simulink model "feedback_3D"  (R2022a)
settings: Solver=VariableStepAuto  StartTime=0.0  StopTime=10.0  RelTol=1e-3
undefined symbols (not defined in the file): A, B, C, F, G, H, K
settings Model: Creator=Orkun  LastModifiedBy=Orkun

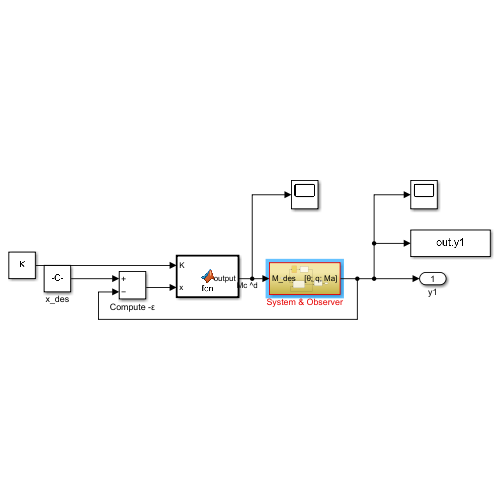
[thumbnail: Simulink's stored preview of the top-level diagram]
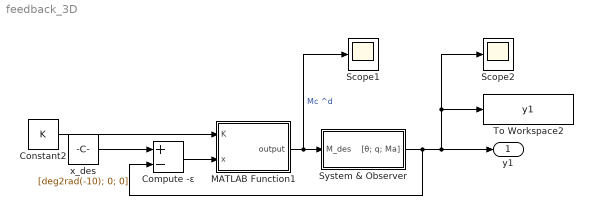
== system feedback_3D ==
  Compute -ε : Sum  Inputs=+-
  Constant2 : Constant  Value=K  VectorParams1D=off
  MATLAB Function1 : MATLAB Function  TreatAsAtomicUnit=on
  Scope1 : Scope
  Scope2 : Scope
  System & Observer : Subsystem
  To Workspace2 : ToWorkspace  VariableName=y1  SaveFormat=Timeseries  SampleTime=-1
  x_des : Constant  Value=[deg2rad(-10); 0; 0]
  y1 : Outport
  wires:
  Compute -ε/1 -> MATLAB Function1/2(x)
  MATLAB Function1/1(output) -> System & Observer/1(M_des), Scope1/1  "Mc ^d"
  Constant2/1 -> MATLAB Function1/1(K)
  x_des/1 -> Compute -ε/1
  System & Observer/1("[θ; q; Ma]") -> Compute -ε/2, Scope2/1, To Workspace2/1, y1/1

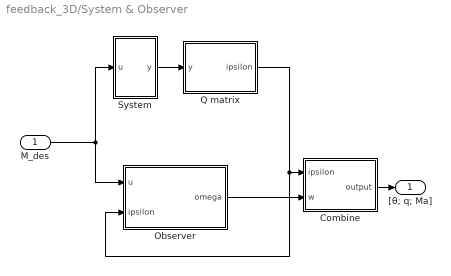
== system feedback_3D/System & Observer ==
  M_des : Inport
  Combine : MATLAB Function  TreatAsAtomicUnit=on
  Observer : Subsystem
  Q matrix : MATLAB Function  TreatAsAtomicUnit=on
  System : Subsystem
  "[θ; q; Ma]" : Outport
  wires:
  M_des/1 -> Observer/1(u), System/1(u)
  Q matrix/1(ipsilon) -> Combine/1(ipsilon), Observer/2(ipsilon)
  Combine/1(output) -> "[θ; q; Ma]"/1
  System/1(y) -> Q matrix/1(y)
  Observer/1(omega) -> Combine/2(w)

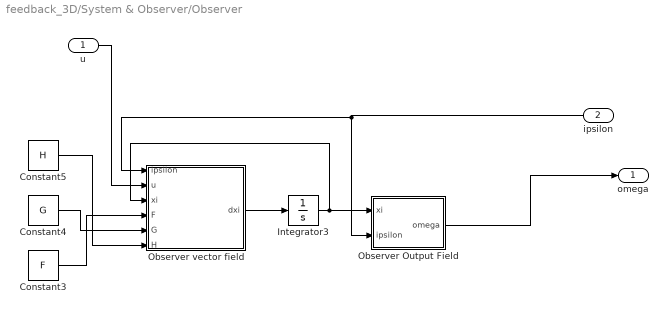
== system feedback_3D/System & Observer/Observer ==
  u : Inport
  ipsilon : Inport  Port=2
  Constant3 : Constant  Value=F
  Constant4 : Constant  Value=G
  Constant5 : Constant  Value=H
  Integrator3 : Integrator  InitialCondition=[0]
  Observer Output Field : MATLAB Function  TreatAsAtomicUnit=on
  Observer vector field : MATLAB Function  TreatAsAtomicUnit=on
  omega : Outport
  wires:
  u/1 -> Observer vector field/2(u)
  Integrator3/1 -> Observer vector field/3(xi), Observer Output Field/1(xi)
  ipsilon/1 -> Observer Output Field/2(ipsilon), Observer vector field/1(ipsilon)
  Constant5/1 -> Observer vector field/6(H)
  Observer Output Field/1(omega) -> omega/1
  Observer vector field/1(dxi) -> Integrator3/1
  Constant4/1 -> Observer vector field/5(G)
  Constant3/1 -> Observer vector field/4(F)

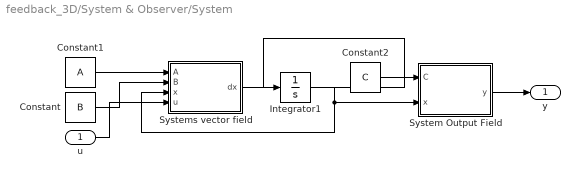
== system feedback_3D/System & Observer/System ==
  u : Inport
  Constant : Constant  Value=B
  Constant1 : Constant  Value=A
  Constant2 : Constant  Value=C
  Integrator1 : Integrator  InitialCondition=[deg2rad(0);0; 0]
  System Output Field : MATLAB Function  TreatAsAtomicUnit=on
  Systems vector field : MATLAB Function  TreatAsAtomicUnit=on
  y : Outport
  wires:
  Systems vector field/1(dx) -> Integrator1/1
  Constant1/1 -> Systems vector field/1(A)
  Constant2/1 -> System Output Field/1(C)
  u/1 -> Systems vector field/4(u)
  Integrator1/1 -> Systems vector field/3(x), System Output Field/2(x)
  System Output Field/1(y) -> y/1
  Constant/1 -> Systems vector field/2(B)

== matlab function feedback_3D/MATLAB Function1 ==
  data: K input; output output; x input
function output = fcn(K, x)

output = K*x;

== matlab function feedback_3D/System & Observer/Combine ==
  data: ipsilon input; output output; w input
function output = fcn(ipsilon, w)

output = [ipsilon;w];

== matlab function feedback_3D/System & Observer/Observer/Observer Output Field ==
  data: xi input; omega output; ipsilon input
function omega = fcn(xi, ipsilon)

L = [0, -0.0475; 0, 2.7];

omega = xi + L*ipsilon;

== matlab function feedback_3D/System & Observer/Observer/Observer vector field ==
  data: ipsilon input; u input; dxi output; xi input; F input; G input; H input
function dxi = fcn(ipsilon,u, xi, F, G, H)
%F = [-16.3046, 0.0475; -967.95, -2.7];
%F = [-16.3046, 0; -967.9500, 0];
%G = [33.3333; 0];
%H = [-0.5621, 0.8753; 31.9507, 40.2480];
%H = [-0.5621, 0.747; 31.9507, 47.5382];


dxi = F*xi + H*ipsilon + G*u;

== matlab function feedback_3D/System & Observer/Q matrix ==
  data: y input; ipsilon output
function ipsilon = fcn(y)

ipsilon = [1, 0; 0, 1]*y;

== matlab function feedback_3D/System & Observer/System/System Output Field ==
  data: C input; x input; y output
function y = fcn(C, x)

%C = [1, 0, 0, 0; 0, 1, 0, 0];
y = C*x;

== matlab function feedback_3D/System & Observer/System/Systems vector field ==
  data: A input; B input; x input; u input; dx output
function dx = fcn(A, B, x, u)

dx = (A*x) + (B*u);
